simulink model "simu_Fuzzy_fuyang"  (R2023a)
settings: Solver=ode4  StartTime=0.0  StopTime=20.0  FixedStep=0.01  RelTol=1e-3  EnableMultiTasking=on
undefined symbols (not defined in the file or in its folder): Test
libraries: fuzblock x1
settings Model: Creator=Administrator  LastModifiedBy=zhs20
settings SolverCC: AlgebraicLoopSolver=TrustRegion
settings DataIOCC: LimitDataPoints=on  SaveFormat=Array  ReturnWorkspaceOutputs=off
settings OptimizationCC: ExpressionDepthLimit=2147483647  LifeSpan=inf
settings DebuggingCC: UnderspecifiedInitializationDetection=Classic  MergeDetectMultiDrivingBlocksExec=none  SolverPrmCheckMsg=warning  UnconnectedInputMsg=warning  UnconnectedOutputMsg=warning  UnconnectedLineMsg=warning  StateNameClashWarn=warning  SFUnexpectedBacktrackingDiag=warning  SFNoUnconditionalDefaultTransitionDiag=warning  SFExecutionAtInitializationDiag=none  ArithmeticOperatorsInVariantConditions=warning
settings HardwareCC: ProdBitPerPointer=32  ProdBitPerSizeT=32  ProdBitPerPtrDiffT=32  ProdLargestAtomicFloat=None  ProdIntDivRoundTo=Undefined  ProdEndianess=Unspecified  ProdWordSize=32  ProdHWDeviceType=32-bit Generic
settings ModelReferenceCC: PropagateSignalLabelsOutOfModel=off
settings SFSimCC: SimUseLocalCustomCode=off  CustomCodeUndefinedFunction=UseInterfaceOnly
settings RTWCC: RTWUseLocalCustomCode=off
settings CodeAppCC: StateflowObjectComments=on
settings GRTTargetCC: TargetLangStandard=C89/C90 (ANSI)
settings ConfigComp: CovMetricSettings=dw  CovSaveCumulativeToWorkspaceVar=on  CovSaveSingleToWorkspaceVar=on  CovExternalEMLEnable=off

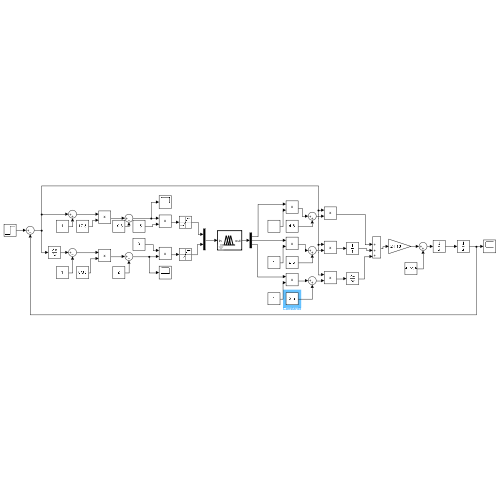
[thumbnail: Simulink's stored preview of the top-level diagram]
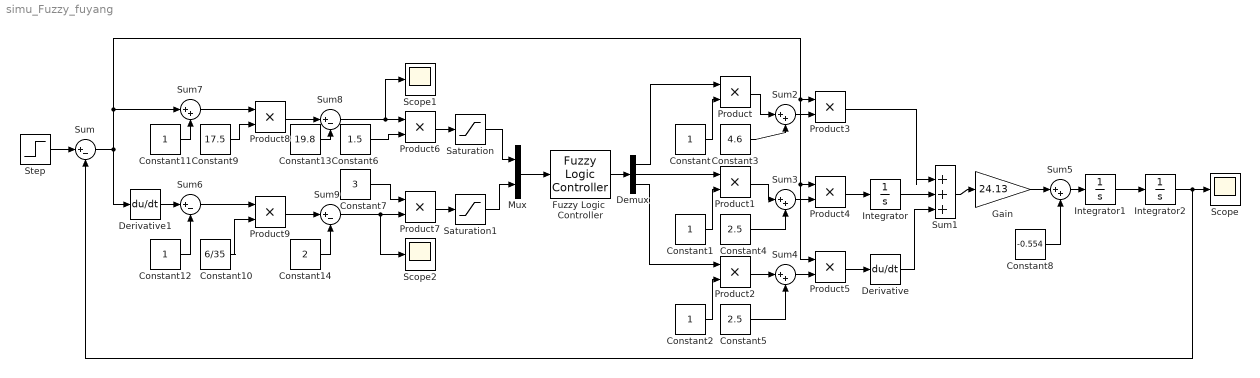
== system simu_Fuzzy_fuyang ==
  Constant{,1..2,11..12} (5 alike) : Constant
  Constant10 : Constant  Value=6/35
  Constant13 : Constant  Value=19.8
  Constant14 : Constant  Value=2
  Constant3 : Constant  Value=4.6
  Constant4 : Constant  Value=2.5
  Constant5 : Constant  Value=2.5
  Constant6 : Constant  Value=1.5
  Constant7 : Constant  Value=3
  Constant8 : Constant  Value=-0.554
  Constant9 : Constant  Value=17.5
  Demux : Demux  Outputs=3
  Derivative : Derivative
  Derivative1 : Derivative
  Fuzzy Logic  Controller : fuzblock/Fuzzy Logic  Controller  FIS=[Test]  OutputSampleNumber=101  DataType=double  FuzzifiedInputs=off  RuleFiringStrengths=off  RuleOutputs=off  AggregatedOutputs=off  SimulateUsing=Interpreted execution  OutOfRangeInputValueMessage=warning  NoRuleFiredMessage=warning  EmptyOutputFuzzySetMessage=warning
  Gain : Gain  Gain=24.13
  Integrator : Integrator
  Integrator1 : Integrator
  Integrator2 : Integrator
  Mux : Mux  Inputs=2
  Product{,1..9} (10 alike) : Product  RndMeth=Zero
  Saturation : Saturate
  Saturation1 : Saturate
  Scope : Scope
  Scope1 : Scope
  Scope2 : Scope
  Step : Step  After=0.3  SampleTime=0
  Sum{,6,8..9} (4 alike) : Sum  Inputs=|+-
  Sum1 : Sum  Inputs=|+++
  Sum{2..5,7} (5 alike) : Sum  Inputs=|++
  wires:
  Sum1/1 -> Gain/1
  Integrator2/1 -> Sum/2, Scope/1
  Step/1 -> Sum/1
  Product4/1 -> Integrator/1
  Product3/1 -> Sum1/1
  Product5/1 -> Derivative/1
  Integrator/1 -> Sum1/2
  Derivative/1 -> Sum1/3
  Mux/1 -> Fuzzy Logic  Controller/1
  Saturation/1 -> Mux/1
  Saturation1/1 -> Mux/2
  Constant1/1 -> Product1/2
  Constant2/1 -> Product2/2
  Fuzzy Logic  Controller/1 -> Demux/1
  Demux/2 -> Product1/1
  Demux/3 -> Product2/1
  Product1/1 -> Sum3/1
  Product2/1 -> Sum4/1
  Product/1 -> Sum2/1
  Constant3/1 -> Sum2/2
  Constant4/1 -> Sum3/2
  Constant5/1 -> Sum4/2
  Sum2/1 -> Product3/2
  Sum3/1 -> Product4/2
  Sum4/1 -> Product5/2
  Product6/1 -> Saturation/1
  Product7/1 -> Saturation1/1
  Sum/1 -> Product5/1, Product4/1, Product3/1, Sum7/1, Derivative1/1
  Gain/1 -> Sum5/1
  Sum5/1 -> Integrator1/1
  Integrator1/1 -> Integrator2/1
  Constant8/1 -> Sum5/2
  Constant7/1 -> Product7/1
  Constant9/1 -> Product8/2
  Sum7/1 -> Product8/1
  Constant12/1 -> Sum6/2
  Derivative1/1 -> Sum6/1
  Constant/1 -> Product/2
  Demux/1 -> Product/1
  Constant6/1 -> Product6/2
  Constant11/1 -> Sum7/2
  Product8/1 -> Sum8/1
  Sum8/1 -> Scope1/1, Product6/1
  Constant13/1 -> Sum8/2
  Sum6/1 -> Product9/1
  Constant10/1 -> Product9/2
  Product9/1 -> Sum9/1
  Sum9/1 -> Scope2/1, Product7/2
  Constant14/1 -> Sum9/2
